simulink model "DC_kas"  (R2015a)
settings: Solver=ode45  StartTime=0.0  StopTime=8  RelTol=1e-3
values from neighbouring files (symbols this model uses):
  D = [1 1]    [DC_PID_IMC.m]    (also in data.mat)
  J = 10    [DC_PID_IMC.m]    (also in DCtest.m; data.mat)
  KE = 8.50    (= 8.5)    [DC_PID_IMC.m]    (also in DCtest.m; data.mat)
  KT = 8.50    (= 8.5)    [DC_PID_IMC.m]    (also in DCtest.m; data.mat)
  Kvi = 2309.4    [DC_PID_IMC.m]    (also in data.mat)
  Kvp = 115.47    [DC_PID_IMC.m]    (also in data.mat)
  La = 0.003    [DC_PID_IMC.m]    (also in DCtest.m; data.mat)
  Ra = 0.15    [DC_PID_IMC.m]    (also in DCtest.m; data.mat)
  TL = 0    [DC_PID_IMC.m]    (also in DCtest.m; data.mat)
undefined symbols (not defined in the file or in its folder): sigbuilder_block
settings Model: Creator=yusuke  LastModifiedBy=yusuke

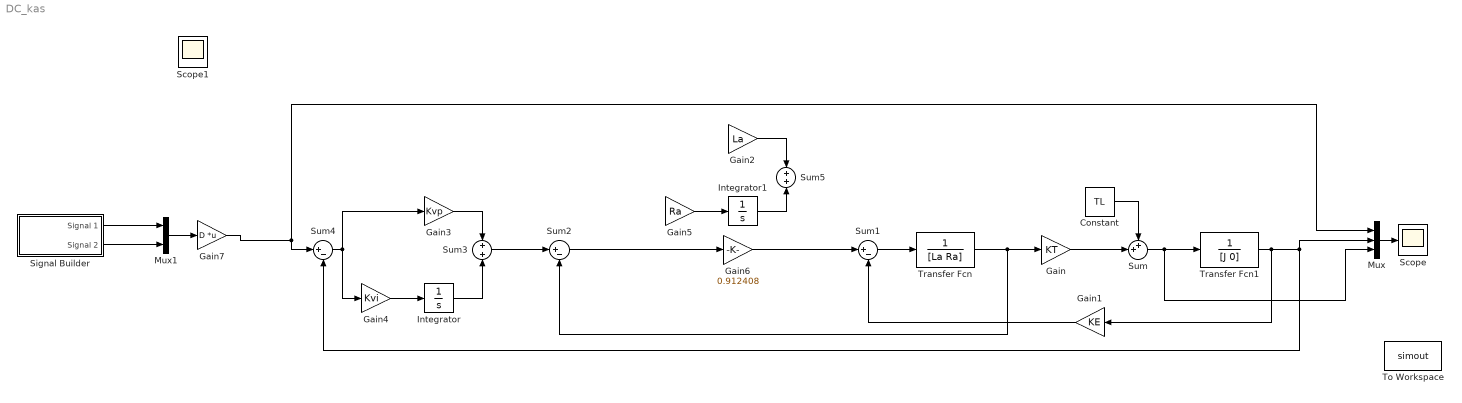
== system DC_kas ==
  Constant : Constant  Value=TL
  Gain : Gain  Gain=KT
  Gain1 : Gain  Gain=KE
  Gain2 : Gain  Gain=La
  Gain3 : Gain  Gain=Kvp
  Gain4 : Gain  Gain=Kvi
  Gain5 : Gain  Gain=Ra
  Gain6 : Gain  Gain=0.912408
  Gain7 : Gain  Gain=D  Multiplication=Matrix(K*u) (u vector)
  Integrator : Integrator
  Integrator1 : Integrator
  Mux : Mux  Inputs=3
  Mux1 : Mux  Inputs=2
  Scope : Scope
      settings: TimeRange=0.5  YMin=-15  YMax=15
  Signal Builder : Subsystem  Tag=STV Subsys  LoadFcn=sigbuilder_block('load',[352.5 -2.25 551.25 401.25 ]);  StartFcn=sigbuilder_block('start');  StopFcn=sigbuilder_block('stop');  ClipboardFcn=sigbuilder_block('clipboard');  mask(Sigbuilder block){}
      mask help: Simulink:masks:SigbuilderBlock_MD
      mask init:
      | if ~strcmp(get_param(bdroot(gcbh),'SimulationStatus'),'stopped') tuvar = sigbuilder_block('maskInit'); end
      settings: CopyFcn=sigbuilder_block('copy');  DeleteFcn=sigbuilder_block('delete');  ModelCloseFcn=sigbuilder_block('modelClose');  PreSaveFcn=sigbuilder_block('preSave');  PauseFcn=sigbuilder_block('pause');  ContinueFcn=sigbuilder_block('continue');  NameChangeFcn=sigbuilder_block('namechange');  OpenFcn=sigbuilder_block('open',[437.6 199.2 550.4 400 ]);  CloseFcn=sigbuilder_block('close');
      mask Display: plot(0, 0, 100, 100,[2, 2, 32, 32, 2], [68, 8, 8, 68, 68],[32, 2], [38, 38], [32, 19, 2],[53, 60, 44], [32, 17, 17, 2],[16, 16, 31, 31]);txt = getActiveGroup(gcbh);text(2, 100, txt,'verticalAlignment', 'top');
  Sum : Sum  Inputs=++|
  Sum1 : Sum  Inputs=|+-
  Sum2 : Sum  Inputs=|+-
  Sum3 : Sum  Inputs=+|+
  Sum4 : Sum  Inputs=|+-
  Sum5 : Sum  Inputs=+|+
  To Workspace : ToWorkspace  VariableName=simout  SaveFormat=Structure With Time  SampleTime=-1
  Transfer Fcn : TransferFcn  Denominator=[La Ra]
  Transfer Fcn1 : TransferFcn  Denominator=[J 0]
  Scope1 : Scope
  wires:
  Transfer Fcn/1 -> Sum2/2, Gain/1
  Gain/1 -> Sum/2
  Constant/1 -> Sum/1
  Sum/1 -> Mux/3, Transfer Fcn1/1
  Transfer Fcn1/1 -> Sum4/2, Mux/2, Gain1/1
  Gain1/1 -> Sum1/2
  Sum1/1 -> Transfer Fcn/1
  Sum3/1 -> Sum2/1
  Gain3/1 -> Sum3/1
  Integrator/1 -> Sum3/2
  Gain4/1 -> Integrator/1
  Sum4/1 -> Gain4/1, Gain3/1
  Gain2/1 -> Sum5/1
  Integrator1/1 -> Sum5/2
  Gain5/1 -> Integrator1/1
  Mux/1 -> Scope/1
  Gain7/1 -> Sum4/1, Mux/1
  Gain6/1 -> Sum1/1
  Sum2/1 -> Gain6/1
  Signal Builder/2(Signal 2) -> Mux1/2
  Mux1/1 -> Gain7/1
  Signal Builder/1(Signal 1) -> Mux1/1
  ? -> To Workspace/1

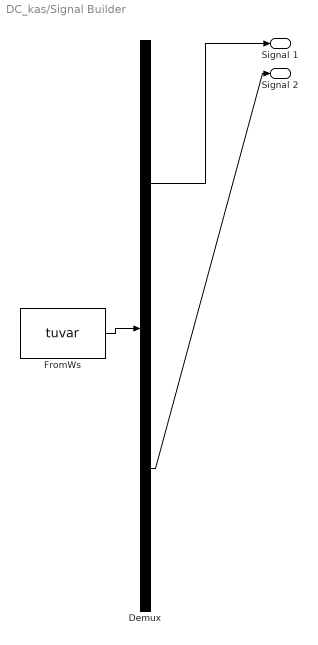
== system DC_kas/Signal Builder ==
  Demux : Demux  Tag=STV Demux  Outputs=2
  FromWs : FromWorkspace  Tag=STV FromWs  VariableName=tuvar  SampleTime=0
      SigBuilderData=|
      | common.afterFinalStr = 'Extrapolate'
      | common.sampleTime = 0
      | dataSet.timeRange = [0 8]
      | dataSet.name = 'Group 1'
      | sbobj.Groups.Name = 'Group 1'
      | sbobj.Groups.Signals(1).Name = 'Signal 1'
      | sbobj.Groups.Signals(1).XData = [0 2 2 8]
      | sbobj.Groups.Signals(1).YData = [500 500 0 0]
      | sbobj.Groups.Signals(2).Name = 'Signal 2'
      | sbobj.Groups.Signals(2).XData = [0 4 4 6 6 8]
      | sbobj.Groups.Signals(2).YData = [0 0 -500 -500 0 0]
      | sbobj.Groups.TimeRange = [0 8]
  Signal 1 : Outport  Tag=STV Outport
  Signal 2 : Outport  Tag=STV Outport  Port=2
  wires:
  Demux/1 -> Signal 1/1
  FromWs/1 -> Demux/1
  Demux/2 -> Signal 2/1
